simulink model "sf_seqrec"  (Simulink 7.6)
settings: Solver=FixedStepDiscrete  StartTime=0.0  StopTime=10.0  RelTol=1e-3
undefined symbols (not defined in the file or in its folder): sigbuilder_block
Description:
  | This demo shows how Mealy and Moore machines can be used in signal processing applications; in this case, for sequence recognition.  In the Moore machine, actions can only be state actions, whereas in the Mealy machine, actions can only be condition actions.
  | 
  | The two Stateflow(R) charts are used to find the sequence 1,2,1,3 in the input signal from Signal Builder.  The status of the sequence recognition is logged in the output variable "state."  If the sequence is found, the variable seqFound is set to 1.  On running the simulation and opening the scopes, notice that the Moore output is delayed by one time step.  This is because the output from a Moore machine is based on the state from the previous time step, and the output from a Mealy machine is based on the state from the previous time step and the current input.
  | 
  | Ref: Digital Design: From Gates to Intelligent Machines, 2006 by Bruce F. Katz
settings Model: Creator=The MathWorks Inc.
settings OptimizationCC: InitFltsAndDblsToZero=on  EfficientMapNaN2IntZero=off  OptimizeModelRefInitCode=on  LifeSpan=1
settings DebuggingCC: SaveWithParameterizedLinksMsg=none  SignalResolutionControl=TryResolveAllWithWarning  StrictBusMsg=Warning
settings SFSimCC: SimParseCustomCode=off
settings RTWCC: SystemTargetFile=ert.tlc  GenCodeOnly=on  TemplateMakefile=ert_default_tmf  Description=Real-Time Workshop Embedded Coder (no auto configuration)  ProcessScript=ert_make_rtw_hook
settings CodeAppCC: IgnoreCustomStorageClasses=off  CustomSymbolStrGlobalVar=$N$M  CustomSymbolStrType=$N$M  CustomSymbolStrFcn=$N$M$F  CustomSymbolStrMacro=$N$M
settings ERTTargetCC: TargetFcnLib=ansi_tfl_tmw.mat  MultiwordLength=2048  GenerateSampleERTMain=on  IncludeMdlTerminateFcn=off  SupportContinuousTime=on  InlinedParameterPlacement=NonHierarchical  ERTCustomFileTemplate=example_file_process.tlc  ConvertIfToSwitch=off

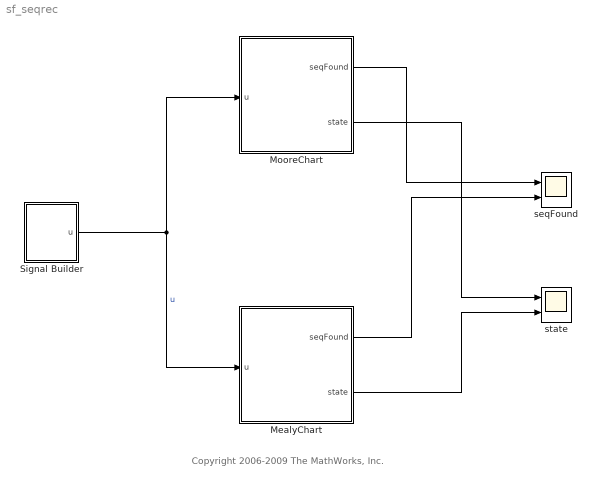
== system sf_seqrec ==
  note: Copyright 2006-2009 The MathWorks, Inc.
  MealyChart : Stateflow chart  TreatAsAtomicUnit=on
  MooreChart : Stateflow chart  TreatAsAtomicUnit=on
  Signal Builder : Subsystem  Tag=STV Subsys  LoadFcn=sigbuilder_block('load');  StartFcn=sigbuilder_block('start');  StopFcn=sigbuilder_block('stop');  ClipboardFcn=sigbuilder_block('clipboard');  mask(Sigbuilder block){}
      mask help: Sigbuilder GUI
      mask init:
      | if ~strcmp(get_param(bdroot(gcbh),'SimulationStatus'),'stopped') tuvar = sigbuilder_block('maskInit'); end
      settings: CopyFcn=sigbuilder_block('copy');  DeleteFcn=sigbuilder_block('delete');  ModelCloseFcn=sigbuilder_block('modelClose');  PreSaveFcn=sigbuilder_block('preSave');  NameChangeFcn=sigbuilder_block('namechange');  OpenFcn=sigbuilder_block('open',[127.5 390 550.5 399.75 ]);  CloseFcn=sigbuilder_block('close');
      mask Display: plot(0,0,100,100,[10,10,40,40,10],[80,20,20,80,80],[40,10],[50,50], [40,27,10],[65,72,56],[40,25,25,10],[28,28,43,43]);
  seqFound : Scope  NumInputPorts=2
      settings: TimeRange=10  YMin=-5~-5  YMax=5~5
  state : Scope  NumInputPorts=2
      settings: TimeRange=10  YMin=-5~-5  YMax=5~5
  wires:
  Signal Builder/1(u) -> MooreChart/1(u), MealyChart/1(u)  "u"
  MooreChart/1(seqFound) -> seqFound/1
  MealyChart/1(seqFound) -> seqFound/2
  MealyChart/2(state) -> state/2
  MooreChart/2(state) -> state/1

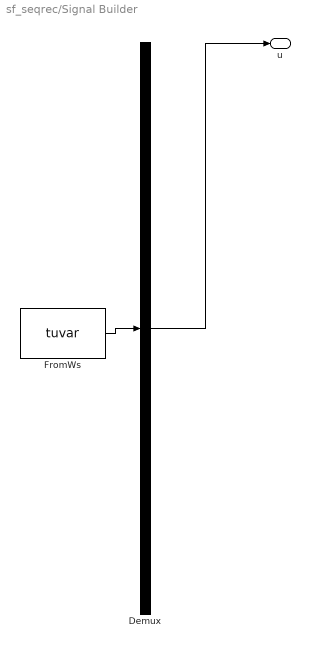
== system sf_seqrec/Signal Builder ==
  Demux : Demux  Tag=STV Demux  Outputs=1
  FromWs : FromWorkspace  Tag=STV FromWs  VariableName=tuvar  SampleTime=0  SigBuilderData=DataTag0  VnvData=DataTag1
      SigBuilderData=|
      | common.afterFinalStr = 'Extrapolate'
      | common.sampleTime = 0
      | dataSet.timeRange = [0 10]
      | dataSet.name = 'Group 1'
      | sbobj.Groups.Name = 'Group 1'
      | sbobj.Groups.Signals.Name = 'u'
      | sbobj.Groups.Signals.XData = [0 0.5 1 1.5 2 2 2.5 3 3 3.5 3.5 4 4 4.5 4.5 5 5 5.5 5.5 6 6 6.5 7 7.5 7.5 8 8 8.5 8.5 9 9 9.5 10]
      | sbobj.Groups.Signals.YData = [1 1 1 1 1 0 0 0 1 1 2 2 1 1 3 3 1 1 2 2 1 1 1 1 2 2 1 1 3 3 1 1 1]
  u : Outport  Tag=STV Outport
  wires:
  Demux/1 -> u/1
  FromWs/1 -> Demux/1

== stateflow chart MooreChart ==
  settings: updateMethod=DISCRETE  sampleTime=0.5  stateMachineType=MOORE_MACHINE  executeAtInitialization=1  initializeOutput=1
  state s0
    state=0;
    seqFound=0;
  state s1
    state=1;
    seqFound=0;
  state s12
    state=2;
  state s121
    state=3;
  state s1213
    state=4;
    seqFound=1;
  s0 -> s1 : [u==1]
  s1 -> s12 [order 1] : [u==2]
  s12 -> s121 [order 1] : [u==1]
  s121 -> s1213 [order 2] : [u==3]
  s1 -> s0 [order 2] : [u!=1]
  s121 -> s12 [order 3] : [u==2]
  (default) -> s0
  s121 -> s1 [order 1] : [u==1]
  s12 -> s0 [order 2]
  s1213 -> s1 [order 1] : [u==1]
  s121 -> s0 [order 4]
  s1213 -> s0 [order 2]
  data: u input double; seqFound output boolean; state output double

== stateflow chart MealyChart ==
  settings: updateMethod=DISCRETE  sampleTime=0.5  stateMachineType=MEALY_MACHINE  executeAtInitialization=1  initializeOutput=1
  state s0
  state s1
  state s12
  state s121
  state s1213
  s0 -> s1 : [u==1]...
      | {state=1;}
  s1 -> s12 [order 1] : [u==2]...
      | {state=2;}
  s12 -> s121 [order 1] : [u==1]...
      | {state=3;}
  s121 -> s1213 [order 2] : [u==3]...
      | {state=4;...
      | seqFound=1;}
  s1 -> s0 [order 2] : [u!=1]{state=0;}
  s121 -> s12 [order 3] : [u==2]...
      | {state=2;}
  s121 -> s1 [order 1] : [u==1]...
      | {state=1;}
  s1213 -> s1 [order 1] : [u==1]...
      | {state=1;...
      | seqFound=0;}
  s12 -> s0 [order 2] : {state=0;}
  s121 -> s0 [order 4] : {state=0;}
  s1213 -> s0 [order 2] : {state=0;...
      | seqFound=0;}
  (default) -> s0
  data: u input double; seqFound output boolean =0; state output double
